simulink model "A4s"  (R2021b)
settings: Solver=VariableStepAuto  StartTime=0.0  StopTime=3  RelTol=1e-3
values from neighbouring files (symbols this model uses):
  A = sn(1)+10    [A4.m]
  B = sn(2)+10    [A4.m]
  C = sn(3)+10    [A4.m]
  D = sn(4)+10    [A4.m]
  F = sn(6)+10    [A4.m]
  G = sn(7)+10    [A4.m]
settings Model: Creator=bryan  LastModifiedBy=bryan

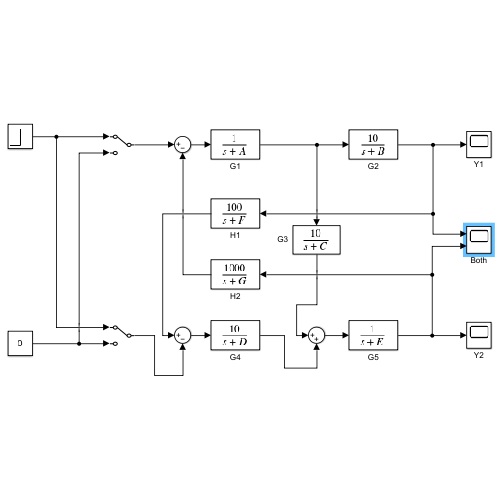
[thumbnail: Simulink's stored preview of the top-level diagram]
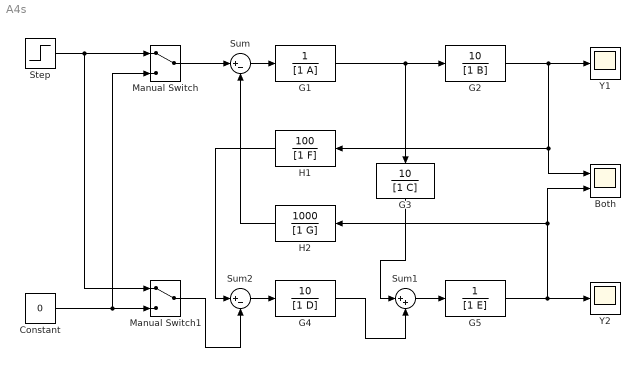
== system A4s ==
  Both : Scope  NumInputPorts=2
  Constant : Constant  Value=0
  G1 : TransferFcn  Denominator=[1 A]  ContinuousStateAttributes="\"G1\""
  G2 : TransferFcn  Numerator=[10]  Denominator=[1 B]
  G3 : TransferFcn  Numerator=[10]  Denominator=[1 C]  ContinuousStateAttributes="\"G3\""
  G4 : TransferFcn  Numerator=[10]  Denominator=[1 D]
  G5 : TransferFcn  Denominator=[1 E]
  H1 : TransferFcn  Numerator=[100]  Denominator=[1 F]
  H2 : TransferFcn  Numerator=[1000]  Denominator=[1 G]
  Manual Switch : ManualSwitch
  Manual Switch1 : ManualSwitch
  Step : Step  Time=0  SampleTime=0
  Sum : Sum  Inputs=|+-
  Sum1 : Sum  Inputs=|++
  Sum2 : Sum  Inputs=|+-
  Y1 : Scope
  Y2 : Scope
  wires:
  Step/1 -> Manual Switch1/1, Manual Switch/1
  Manual Switch/1 -> Sum/1
  Sum/1 -> G1/1
  G1/1 -> G2/1, G3/1
  G2/1 -> Both/1, H1/1, Y1/1
  G3/1 -> Sum1/1
  Constant/1 -> Manual Switch/2, Manual Switch1/2
  Manual Switch1/1 -> Sum2/2
  H1/1 -> Sum2/1
  Sum2/1 -> G4/1
  G4/1 -> Sum1/2
  Sum1/1 -> G5/1
  G5/1 -> Y2/1, Both/2, H2/1
  H2/1 -> Sum/2
